simulink model "MPC"  (R2013a)
settings: Solver=ode45  StartTime=0.0  StopTime=24  RelTol=1e-3
values from neighbouring files (symbols this model uses):
  amp = data.Weighting    [MPCinit.m]
  c = 1005.4    [MPCinit.m]    (also in qp.m)
  C_heater = 20    [MPCinit.m]
  ComfortTemp = str2double(data.ComfortTemp)    [MPCinit.m]
  M = (lenHouse*widHouse*htHouse+tan(pitRoof)*widHouse*lenHouse)*densAir    [MPCinit.m]    (also in qp.m)
  Mdot = 3600*0.2    (= 720)    [MPCinit.m]    (also in qp.m)
  Req = 1/K_eq    [MPCinit.m]
  T_init = averageTemp    [MPCinit.m]
undefined symbols (not defined in the file or in its folder): magnitude
settings Model: Creator=majachar  LastModifiedBy=cjrorvik
settings SolverCC: AlgebraicLoopSolver=LineSearch
settings DataIOCC: LimitDataPoints=off  SignalLoggingSaveFormat=ModelDataLogs
settings DebuggingCC: MultiTaskDSMMsg=warning  MultiTaskCondExecSysMsg=none  StateNameClashWarn=none  StrictBusMsg=None
settings RTWCC: IncludeERTFirstTime=on

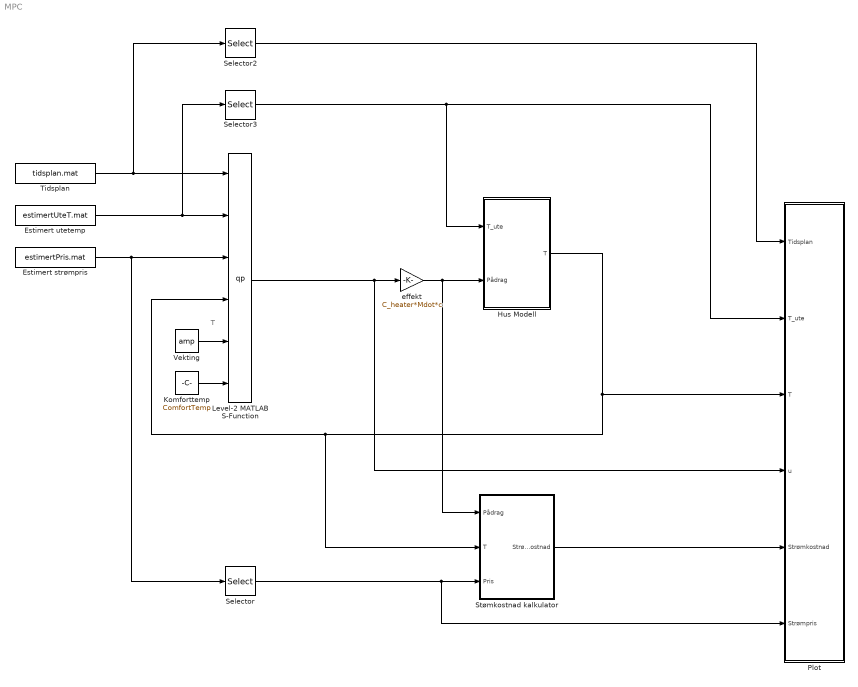
== system MPC ==
  note: T
  Estimert strømpris : FromFile  FileName=estimertPris.mat  SampleTime=0
  Estimert utetemp : FromFile  FileName=estimertUteT.mat  SampleTime=0
  Hus Modell : Subsystem
  Komforttemp : Constant  Value=ComfortTemp
  Level-2 MATLAB S-Function : M-S-Function  FunctionName=qp
  Plot : Subsystem
  Selector : Selector  InputPortWidth=24  IndexOptions=Index vector (dialog)  Indices=[1]  OutputSizes=1
  Selector2 : Selector  InputPortWidth=24  IndexOptions=Index vector (dialog)  Indices=[1]  OutputSizes=1
  Selector3 : Selector  InputPortWidth=24  IndexOptions=Index vector (dialog)  Indices=[1]  OutputSizes=1
  "Stømkostnad kalkulator " : Subsystem
  Tidsplan : FromFile  FileName=tidsplan.mat  SampleTime=0
  Vekting : Constant  Value=amp
  effekt : Gain  Gain=C_heater*Mdot*c
  wires:
  Hus Modell/1(T) -> "Stømkostnad kalkulator "/2("T "), Level-2 MATLAB S-Function/4, Plot/3(T)
  effekt/1 -> Hus Modell/2(Pådrag), "Stømkostnad kalkulator "/1(Pådrag)
  Estimert utetemp/1 -> Level-2 MATLAB S-Function/2, Selector3/1
  Estimert strømpris/1 -> Selector/1, Level-2 MATLAB S-Function/3
  Tidsplan/1 -> Level-2 MATLAB S-Function/1, Selector2/1
  Selector/1 -> "Stømkostnad kalkulator "/3(Pris), Plot/6(Strømpris)
  Selector3/1 -> Hus Modell/1(T_ute), Plot/2(T_ute)
  Vekting/1 -> Level-2 MATLAB S-Function/5
  Selector2/1 -> Plot/1("Tidsplan ")
  "Stømkostnad kalkulator "/1("Strømkostnad ") -> Plot/5(Strømkostnad)
  Level-2 MATLAB S-Function/1 -> Plot/4(u), effekt/1
  Komforttemp/1 -> Level-2 MATLAB S-Function/6

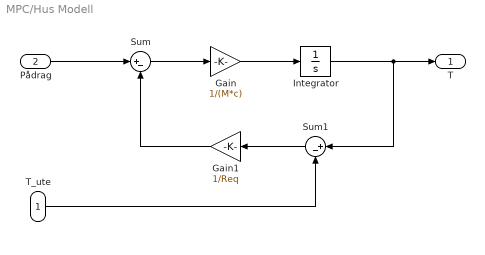
== system MPC/Hus Modell ==
  T_ute : Inport
  Pådrag : Inport  Port=2
  Gain : Gain  Gain=1/(M*c)
  Gain1 : Gain  Gain=1/Req
  Integrator : Integrator  InitialCondition=T_init
  Sum : Sum  Inputs=|+-
  Sum1 : Sum  Inputs=|+-
  T : Outport
  wires:
  Integrator/1 -> Sum1/1, T/1
  Gain/1 -> Integrator/1
  Pådrag/1 -> Sum/1
  Gain1/1 -> Sum/2
  Sum/1 -> Gain/1
  Sum1/1 -> Gain1/1
  T_ute/1 -> Sum1/2

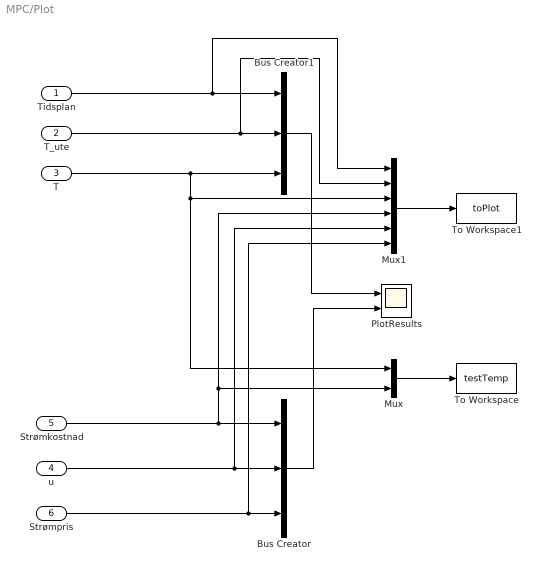
== system MPC/Plot ==
  "Tidsplan " : Inport
  T_ute : Inport  Port=2
  T : Inport  Port=3
  u : Inport  Port=4
  Strømkostnad : Inport  Port=5
  Strømpris : Inport  Port=6
  Bus Creator : BusCreator  Inputs=3
  Bus Creator1 : BusCreator  Inputs=3
  Mux : Mux  Inputs=2
  Mux1 : Mux  Inputs=6
  PlotResults : Scope  NumInputPorts=2
      settings: TimeRange=6  YMin=-5~0  YMax=22.5~21  SaveName=a
  To Workspace : ToWorkspace  VariableName=testTemp  SampleTime=-1
  To Workspace1 : ToWorkspace  VariableName=toPlot  SampleTime=-1  SaveFormat=Structure With Time
  wires:
  Bus Creator/1 -> PlotResults/2
  "Tidsplan "/1 -> Mux1/1, Bus Creator1/1
  Bus Creator1/1 -> PlotResults/1
  Mux/1 -> To Workspace/1
  Mux1/1 -> To Workspace1/1
  Strømkostnad/1 -> Mux1/4, Mux/2, Bus Creator/1
  T/1 -> Mux/1, Mux1/3, Bus Creator1/3
  Strømpris/1 -> Mux1/6, Bus Creator/3
  u/1 -> Mux1/5, Bus Creator/2
  T_ute/1 -> Mux1/2, Bus Creator1/2

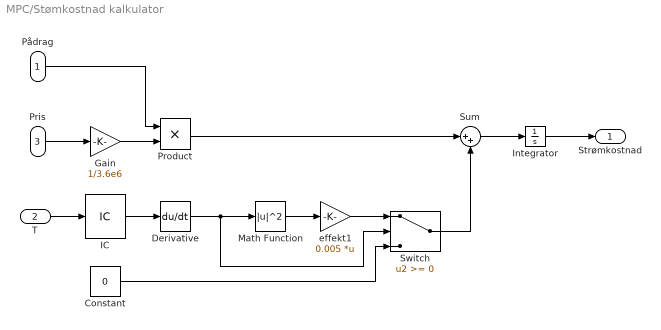
== system MPC/Stømkostnad kalkulator  ==
  Pådrag : Inport
  "T " : Inport  Port=2
  Pris : Inport  Port=3
  Constant : Constant  Value=0
  Derivative : Derivative  CoefficientInTFapproximation=1
  Gain : Gain  Gain=1/3.6e6
  IC : InitialCondition  Value=T_init  SampleTime=1
  Integrator : Integrator
  Math Function : Math  Operator=magnitude^2  OutMax=1  SaturateOnIntegerOverflow=on
  Product : Product
  Sum : Sum  Inputs=|++
  Switch : Switch  OutMax=1
  effekt1 : Gain  Gain=0.005  Multiplication=Matrix(K*u)
  "Strømkostnad " : Outport
  wires:
  Gain/1 -> Product/2
  Math Function/1 -> effekt1/1
  Pådrag/1 -> Product/1
  Pris/1 -> Gain/1
  "T "/1 -> IC/1
  effekt1/1 -> Switch/1
  Constant/1 -> Switch/3
  IC/1 -> Derivative/1
  Derivative/1 -> Switch/2, Math Function/1
  Sum/1 -> Integrator/1
  Switch/1 -> Sum/2
  Product/1 -> Sum/1
  Integrator/1 -> "Strømkostnad "/1
